simulink model "sim_proj1_1"  (R2022a)
settings: Solver=VariableStepAuto  StartTime=0.0  StopTime=1000  RelTol=1e-3
values from neighbouring files (symbols this model uses):
  Ad = sysd.a    [main_proj1.m]    (also in main_proj1_cheese.m)
  Bd = sysd.b    [main_proj1.m]    (also in main_proj1_cheese.m)
  C = eye(4)    [main_proj1.m]    (also in main_proj1_cheese.m = [1 1 0 0)
  D = zeros(4,1)    [main_proj1.m]    (also in main_proj1_cheese.m)
  sample = 1    [main_proj1.m]    (also in main_proj1_cheese.m)
  x_zero = [-0.1,0.1,0.2,-0.2]'    [main_proj1.m]    (also in main_proj1_cheese.m)
undefined symbols (not defined in the file or in its folder): K
libraries: dspsrcs4 x3
settings Model: Creator=tikyn  LastModifiedBy=tikyn

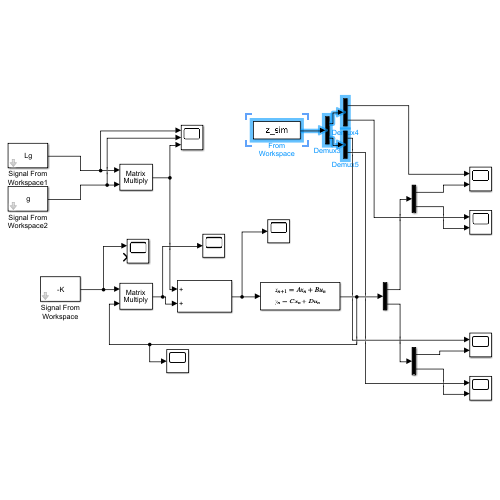
[thumbnail: Simulink's stored preview of the top-level diagram]
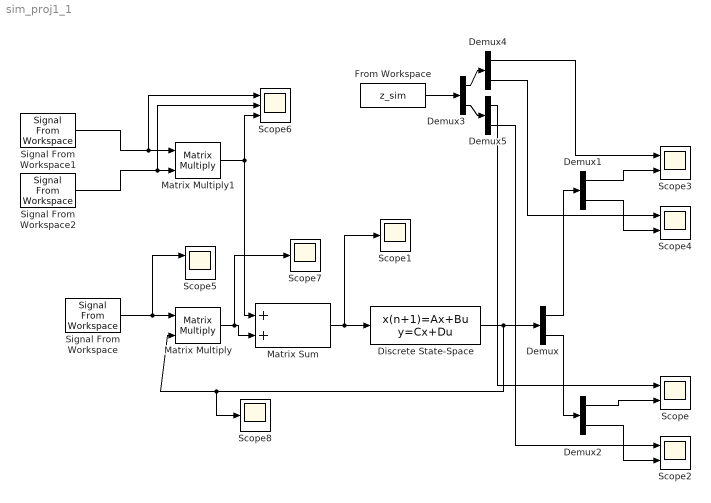
== system sim_proj1_1 ==
  Demux{,1..5} (6 alike) : Demux  Outputs=2
  Discrete State-Space : DiscreteStateSpace  A=Ad  B=Bd  C=C  D=D  InitialCondition=x_zero  SampleTime=sample
  From Workspace : FromWorkspace  VariableName=z_sim  SampleTime=1
  Matrix Sum : Sum
  Matrix Multiply : Product  Multiplication=Matrix(*)
  Matrix Multiply1 : Product  Multiplication=Matrix(*)
  Scope{,2..5} (5 alike) : Scope  NumInputPorts=2
  Scope1 : Scope
  Scope6 : Scope  NumInputPorts=3
  Scope7 : Scope
  Scope8 : Scope
  Signal From Workspace : dspsrcs4/Signal From Workspace  X=-K  Ts=1  nsamps=1  OutputAfterFinalValue=Setting to zero  ignoreOrWarnInputAndFrameLengths=off  OutputFrames=off
  Signal From Workspace1 : dspsrcs4/Signal From Workspace  X=Lg  Ts=1  nsamps=1  OutputAfterFinalValue=Setting to zero  ignoreOrWarnInputAndFrameLengths=off  OutputFrames=off
  Signal From Workspace2 : dspsrcs4/Signal From Workspace  X=g  Ts=1  nsamps=1  OutputAfterFinalValue=Setting to zero  ignoreOrWarnInputAndFrameLengths=off  OutputFrames=off
  wires:
  Discrete State-Space/1 -> Demux/1, Scope8/1, Matrix Multiply/2
  Matrix Multiply/1 -> Scope7/1, Matrix Sum/2
  Matrix Sum/1 -> Discrete State-Space/1, Scope1/1
  Signal From Workspace/1 -> Scope5/1, Matrix Multiply/1
  Signal From Workspace1/1 -> Scope6/1, Matrix Multiply1/1
  Signal From Workspace2/1 -> Scope6/2, Matrix Multiply1/2
  Matrix Multiply1/1 -> Matrix Sum/1, Scope6/3
  Demux/1 -> Demux1/1
  Demux/2 -> Demux2/1
  Demux2/2 -> Scope2/2
  Demux2/1 -> Scope/2
  Demux1/1 -> Scope3/2
  Demux1/2 -> Scope4/2
  From Workspace/1 -> Demux3/1
  Demux3/2 -> Demux5/1
  Demux3/1 -> Demux4/1
  Demux4/1 -> Scope3/1
  Demux4/2 -> Scope4/1
  Demux5/1 -> Scope/1
  Demux5/2 -> Scope2/1
